simulink model "actoac"  (R2024a)
settings: Solver=ode23s  StartTime=0.0  StopTime=0.2  MaxStep=1e-5  MinStep=1e-5  RelTol=1e-3  AbsTol=1e-5
undefined symbols (not defined in the file): aa, de, L
libraries: spsThyristorLib x8, spsCurrentMeasurementLib x3, simulink x2, dspswit3 x2, spsVoltageMeasurementLib x2, dspsigops x2, spsACVoltageSourceLib x1, spsSeriesRLCBranchLib x1, sps_lib x1
settings Model: Creator=arian  LastModifiedBy=arian
settings SolverCC: ZeroCrossAlgorithm=Adaptive
settings DebuggingCC: IgnoredZcDiagnostic=none

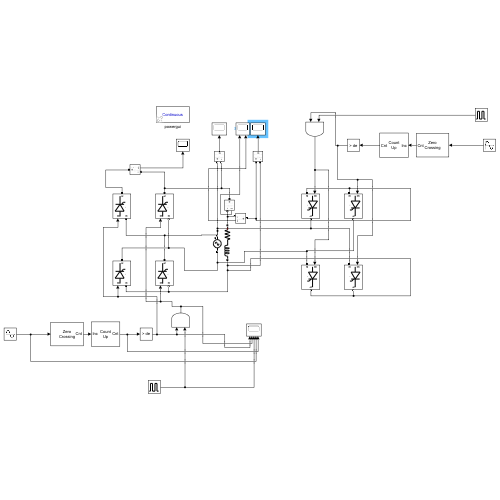
[thumbnail: Simulink's stored preview of the top-level diagram]
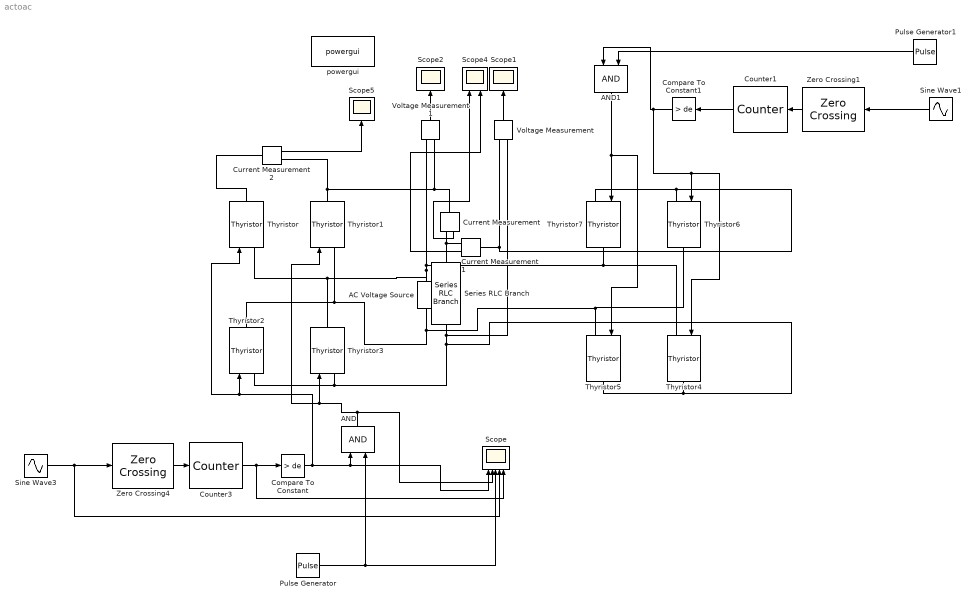
== system actoac ==
  AC Voltage Source : spsACVoltageSourceLib/AC Voltage Source  Amplitude=1  Phase=0  Frequency=50  SampleTime=0  Measurements=None  BusType=swing  Pref=10e3  Qref=0  Qmin=-inf  Qmax=+inf
  AND : Logic  IconShape=distinctive  AllPortsSameDT=off  OutDataTypeStr=boolean
  AND1 : Logic  IconShape=distinctive  AllPortsSameDT=off  OutDataTypeStr=boolean
  Compare To Constant : simulink/Logic and Bit Operations/Compare To Constant  relop=>  const=de  OutDataTypeStr=boolean
  Compare To Constant1 : simulink/Logic and Bit Operations/Compare To Constant  relop=>  const=de  OutDataTypeStr=boolean
  Counter1 : dspswit3/Counter  Direction=Up  CountEvent=Non-zero sample  CounterSize=User defined  MaxCount=2*de-1  InitialCount=de  Output=Count  HitValue=1  ResetInput=off  SamplesPerFrame=1  Ts=1  CntDtype=int8  HitDtype=Logical
  Counter3 : dspswit3/Counter  Direction=Up  CountEvent=Non-zero sample  CounterSize=User defined  MaxCount=2*de-1  InitialCount=0  Output=Count  HitValue=1  ResetInput=off  SamplesPerFrame=1  Ts=1  CntDtype=int8  HitDtype=Logical
  Current Measurement : spsCurrentMeasurementLib/Current Measurement  PhasorSimulation=off  OutputType=Complex  PSBequivalent=0
  Current Measurement1 : spsCurrentMeasurementLib/Current Measurement  PhasorSimulation=off  OutputType=Complex  PSBequivalent=0
  Current Measurement2 : spsCurrentMeasurementLib/Current Measurement  PhasorSimulation=off  OutputType=Complex  PSBequivalent=0
  Pulse Generator : DiscretePulseGenerator  PulseType=Time based  Period=0.01  PulseWidth=5  PhaseDelay=aa
  Pulse Generator1 : DiscretePulseGenerator  PulseType=Time based  Period=0.01  PulseWidth=5  PhaseDelay=aa
  Scope : Scope  NumInputPorts=5
  Scope1 : Scope
  Scope2 : Scope
  Scope4 : Scope  NumInputPorts=2
  Scope5 : Scope
  Series RLC Branch : spsSeriesRLCBranchLib/Series RLC Branch  LConnTagsString=__new0  RConnTagsString=__new0  BranchType=RL  Resistance=1  Inductance=L  SetiL0=off  InitialCurrent=0  Capacitance=1e-6  Setx0=off  InitialVoltage=0  Measurements=None
  Sine Wave1 : Sin  Amplitude=10  Frequency=50*(2*pi)  SampleTime=0
  Sine Wave3 : Sin  Amplitude=10  Frequency=50*(2*pi)  SampleTime=0
  Thyristor{,1..7} (8 alike) : spsThyristorLib/Thyristor  Ron=0  Lon=0  Vf=0  IC=0  Rs=inf  Cs=inf  Measurements=off
  Voltage Measurement : spsVoltageMeasurementLib/Voltage Measurement  PhasorSimulation=off  OutputType=Complex  PSBequivalent=0
  Voltage Measurement1 : spsVoltageMeasurementLib/Voltage Measurement  PhasorSimulation=off  OutputType=Complex  PSBequivalent=0
  Zero Crossing1 : dspsigops/Zero Crossing  InputProcessing=Columns as channels (frame based)
  Zero Crossing4 : dspsigops/Zero Crossing  InputProcessing=Columns as channels (frame based)
  powergui : sps_lib/powergui  Priority=1  SimulationMode=Continuous  SampleTime=50e-6  frequency=60  Iterations=50  frequencyindice=50  Pbase=100e6  ErrMax=1e-4  UnitsV=kV  UnitsW=MW  buscounter=0  FunctionMessages=off  echomessages=off  EnableUseOfTLC=off  CurrentSourceSwitches=off  DisableSnubberDevices=off  DisableRonSwitches=off  DisableVfSwitches=off  DisplayEquations=off  AutomaticDiscreteSolvers=off  SolverType=Tustin/Backward Euler (TBE)  Interpol=off  ExternalGateDelay=off  methode=off  Ts=100  x0status=blocks  SPID=on  SwTol=0  HookPort=off  NonlinearTolerance=1e-4  nMaxIteration=100  ContinueOnMaxIteration=off  RestoreLinks=warning  ResistiveCurrentMeasurement=off  Frange=[0:2:500]  Ylog=off  Xlog=on  ShowGrid=off  save=off  variable=ZData  structure=0  ZoomFFT=off  StartTime=0.0  cycles=1  DisplayStyle=1  fundamental=60  FreqAxis=off  MaxFrequency=1000  frequencyindicesteady=1  RmsSteady=1  display=off
  wires:
  Voltage Measurement/1 -> Scope1/1
  Zero Crossing4/1 -> Counter3/1
  Sine Wave3/1 -> Scope/4, Zero Crossing4/1
  Counter3/1 -> Scope/5, Compare To Constant/1
  Counter1/1 -> Compare To Constant1/1
  Sine Wave1/1 -> Zero Crossing1/1
  Zero Crossing1/1 -> Counter1/1
  Current Measurement/1 -> Scope4/1
  Current Measurement1/1 -> Scope4/2
  Current Measurement2/1 -> Scope5/1
  Voltage Measurement1/1 -> Scope2/1
  Pulse Generator/1 -> Scope/3, AND/2
  Compare To Constant/1 -> Scope/1, AND/1, Thyristor/1, Thyristor2/1
  AND/1 -> Thyristor1/1, Thyristor3/1, Scope/2
  Compare To Constant1/1 -> AND1/1, Thyristor4/1, Thyristor6/1
  Pulse Generator1/1 -> AND1/2
  AND1/1 -> Thyristor5/1, Thyristor7/1
  connections:
  AC Voltage Source/LConn1 -- Thyristor6/RConn1 -- Thyristor5/LConn1 -- Thyristor2/RConn1 -- Thyristor1/LConn1
  Series RLC Branch/LConn1 -- Current Measurement1/RConn1 -- Current Measurement/RConn1
  Voltage Measurement1/LConn1 -- Thyristor4/LConn1 -- Thyristor7/RConn1 -- Thyristor/LConn1 -- Thyristor3/RConn1 -- AC Voltage Source/RConn1
  Thyristor4/RConn1 -- Thyristor5/RConn1 -- Thyristor3/LConn1 -- Thyristor2/LConn1 -- Voltage Measurement/LConn2 -- Series RLC Branch/RConn1
  Thyristor/RConn1 -- Current Measurement2/LConn1
  Thyristor6/LConn1 -- Thyristor7/LConn1 -- Voltage Measurement/LConn1 -- Current Measurement1/LConn1
  Current Measurement/LConn1 -- Current Measurement2/RConn1 -- Thyristor1/RConn1 -- Voltage Measurement1/LConn2
